simulink model "Parachute1DOF"  (R2022a)
settings: Solver=VariableStepAuto  StartTime=0.0  StopTime=60  RelTol=1e-3
values from neighbouring files (symbols this model uses):
  g = 9.81    [initialize_6DoF.m]
undefined symbols (not defined in the file or in its folder): alt, Cd, density, mass, Pra
settings Model: Creator=ben60  LastModifiedBy=ben60

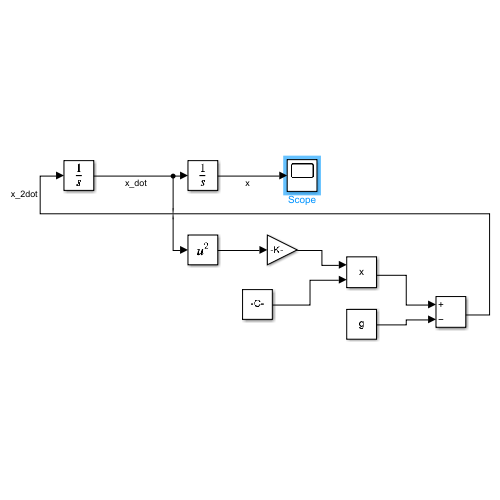
[thumbnail: Simulink's stored preview of the top-level diagram]
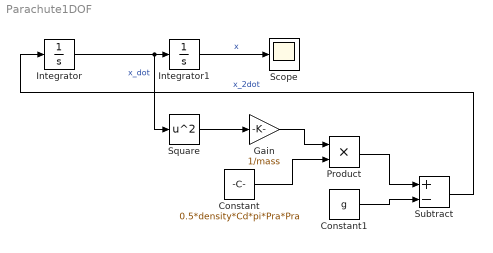
== system Parachute1DOF ==
  Constant : Constant  Value=0.5*density*Cd*pi*Pra*Pra
  Constant1 : Constant  Value=g
  Gain : Gain  Gain=1/mass
  Integrator : Integrator
  Integrator1 : Integrator  InitialCondition=alt
  Product : Product
  Scope : Scope
  Square : Math  Operator=square
  Subtract : Sum  Inputs=+-
  wires:
  Integrator/1 -> Square/1, Integrator1/1  "x_dot"
  Subtract/1 -> Integrator/1  "x_2dot"
  Integrator1/1 -> Scope/1  "x"
  Square/1 -> Gain/1
  Gain/1 -> Product/1
  Constant/1 -> Product/2
  Constant1/1 -> Subtract/2
  Product/1 -> Subtract/1
